simulink model "Batterieersatzschaltbild"  (R2020a)
settings: Solver=VariableStepAuto  StartTime=0.0  StopTime=20  RelTol=1e-3
PreLoadFcn:
  | SubsystemVerbraucherwiderstand = Simulink.Variant('Mode == 1');
  | SubsystemVerbraucherleistung = Simulink.Variant('Mode == 2')
undefined symbols (not defined in the file or in its folder): c_Mo, J_T, L, M_L, Pges, R_A, R_i, Rv, U_b0
settings Model: Creator=ferdi  LastModifiedBy=ferdi

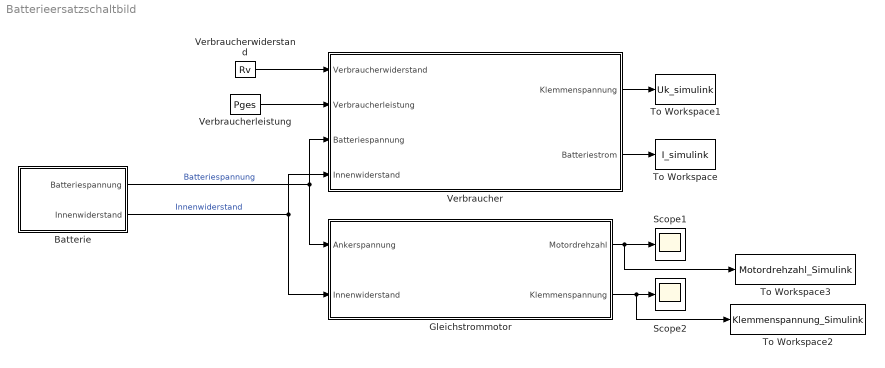
== system Batterieersatzschaltbild ==
  Batterie : Subsystem
      mask Display: image('$imagefile'); % Use "Edit Image" on toolstrip to change.
  Gleichstrommotor : Subsystem
  Scope1 : Scope
  Scope2 : Scope
  To Workspace : ToWorkspace  VariableName=I_simulink  SaveFormat=Timeseries  SampleTime=-1
  To Workspace1 : ToWorkspace  VariableName=Uk_simulink  SaveFormat=Timeseries  SampleTime=-1
  To Workspace2 : ToWorkspace  VariableName=Klemmenspannung_Simulink  SaveFormat=Timeseries  SampleTime=-1
  To Workspace3 : ToWorkspace  VariableName=Motordrehzahl_Simulink  SaveFormat=Timeseries  SampleTime=-1
  Verbraucher : Subsystem  Variant=on
  Verbraucherleistung : Constant  Value=Pges
  Verbraucherwiderstand : Constant  Value=Rv
  wires:
  Gleichstrommotor/1(Motordrehzahl) -> To Workspace3/1, Scope1/1
  Verbraucher/2(Batteriestrom) -> To Workspace/1
  Verbraucher/1(Klemmenspannung) -> To Workspace1/1
  Verbraucherleistung/1 -> Verbraucher/2(Verbraucherleistung)
  Verbraucherwiderstand/1 -> Verbraucher/1(Verbraucherwiderstand)
  Batterie/2(Innenwiderstand) -> Gleichstrommotor/2(Innenwiderstand), Verbraucher/4(Innenwiderstand)  "Innenwiderstand"
  Batterie/1(Batteriespannung) -> Gleichstrommotor/1(Ankerspannung), Verbraucher/3(Batteriespannung)  "Batteriespannung"
  Gleichstrommotor/2(Klemmenspannung) -> To Workspace2/1, Scope2/1

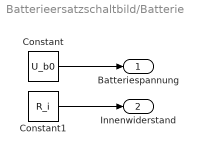
== system Batterieersatzschaltbild/Batterie ==
  Constant : Constant  Value=U_b0
  Constant1 : Constant  Value=R_i
  Batteriespannung : Outport
  Innenwiderstand : Outport  Port=2
  wires:
  Constant/1 -> Batteriespannung/1
  Constant1/1 -> Innenwiderstand/1

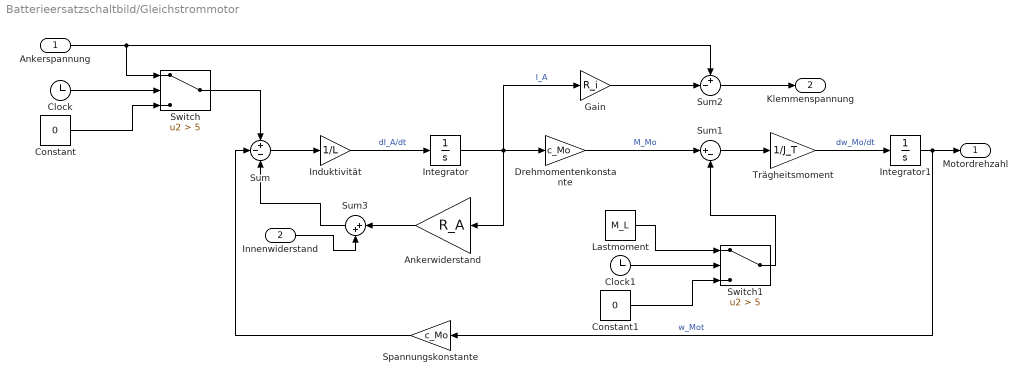
== system Batterieersatzschaltbild/Gleichstrommotor ==
  Ankerspannung : Inport
  Innenwiderstand : Inport  Port=2
  Ankerwiderstand : Gain  Gain=R_A
  Clock : Clock
  Clock1 : Clock
  Constant : Constant  Value=0
  Constant1 : Constant  Value=0
  Drehmomentenkonstante : Gain  Gain=c_Mo
  Gain : Gain  Gain=R_i
  Induktivität : Gain  Gain=1/L
  Integrator : Integrator
  Integrator1 : Integrator
  Lastmoment : Constant  Value=M_L
  Spannungskonstante : Gain  Gain=c_Mo
  Sum : Sum  Inputs=+--
  Sum1 : Sum  Inputs=|+-
  Sum2 : Sum  Inputs=+-|
  Sum3 : Sum  Inputs=|++
  Switch : Switch  Criteria=u2 > Threshold  Threshold=5
  Switch1 : Switch  Criteria=u2 > Threshold  Threshold=5
  Trägheitsmoment : Gain  Gain=1/J_T
  Motordrehzahl : Outport
  Klemmenspannung : Outport  Port=2
  wires:
  Constant/1 -> Switch/3
  Integrator1/1 -> Motordrehzahl/1, Spannungskonstante/1  "w_Mot"
  Drehmomentenkonstante/1 -> Sum1/1  "M_Mo"
  Sum/1 -> Induktivität/1
  Trägheitsmoment/1 -> Integrator1/1  "dw_Mo/dt"
  Switch/1 -> Sum/1
  Ankerspannung/1 -> Switch/1, Sum2/1
  Sum2/1 -> Klemmenspannung/1
  Gain/1 -> Sum2/2
  Clock/1 -> Switch/2
  Lastmoment/1 -> Switch1/1
  Spannungskonstante/1 -> Sum/2
  Induktivität/1 -> Integrator/1  "dI_A/dt"
  Sum1/1 -> Trägheitsmoment/1
  Integrator/1 -> Gain/1, Drehmomentenkonstante/1, Ankerwiderstand/1  "I_A"
  Clock1/1 -> Switch1/2
  Constant1/1 -> Switch1/3
  Switch1/1 -> Sum1/2
  Ankerwiderstand/1 -> Sum3/1
  Sum3/1 -> Sum/3
  Innenwiderstand/1 -> Sum3/2

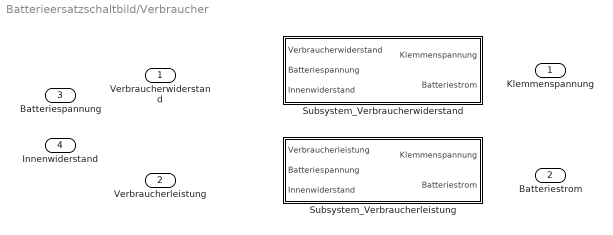
== system Batterieersatzschaltbild/Verbraucher ==
  Verbraucherwiderstand : Inport
  Verbraucherleistung : Inport  Port=2
  Batteriespannung : Inport  Port=3
  Innenwiderstand : Inport  Port=4
  Subsystem_Verbraucherleistung : Subsystem  VariantControl=SubsystemVerbraucherleistung
  Subsystem_Verbraucherwiderstand : Subsystem  VariantControl=SubsystemVerbraucherwiderstand
  Klemmenspannung : Outport
  Batteriestrom : Outport  Port=2

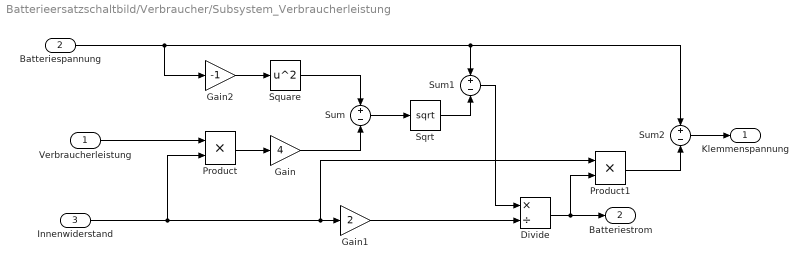
== system Batterieersatzschaltbild/Verbraucher/Subsystem_Verbraucherleistung ==
  Verbraucherleistung : Inport
  Batteriespannung : Inport  Port=2
  Innenwiderstand : Inport  Port=3
  Divide : Product  Inputs=*/
  Gain : Gain  Gain=4
  Gain1 : Gain  Gain=2
  Gain2 : Gain  Gain=-1
  Product : Product
  Product1 : Product
  Sqrt : Sqrt  SaturateOnIntegerOverflow=on
  Square : Math  Operator=square  SaturateOnIntegerOverflow=on
  Sum : Sum  Inputs=+-
  Sum1 : Sum  Inputs=+-
  Sum2 : Sum  Inputs=+-
  Klemmenspannung : Outport
  Batteriestrom : Outport  Port=2
  wires:
  Sum2/1 -> Klemmenspannung/1
  Product1/1 -> Sum2/2
  Sum1/1 -> Divide/1
  Gain1/1 -> Divide/2
  Product/1 -> Gain/1
  Gain/1 -> Sum/2
  Sqrt/1 -> Sum1/2
  Sum/1 -> Sqrt/1
  Square/1 -> Sum/1
  Gain2/1 -> Square/1
  Verbraucherleistung/1 -> Product/1
  Innenwiderstand/1 -> Gain1/1, Product1/1, Product/2
  Batteriespannung/1 -> Sum1/1, Sum2/1, Gain2/1
  Divide/1 -> Batteriestrom/1, Product1/2

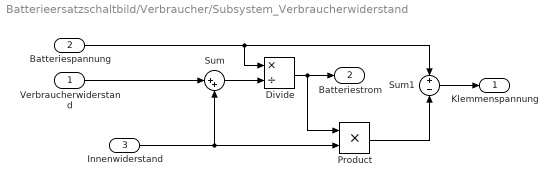
== system Batterieersatzschaltbild/Verbraucher/Subsystem_Verbraucherwiderstand ==
  Verbraucherwiderstand : Inport
  Batteriespannung : Inport  Port=2
  Innenwiderstand : Inport  Port=3
  Divide : Product  Inputs=*/
  Product : Product
  Sum : Sum  Inputs=|++
  Sum1 : Sum  Inputs=+-
  Klemmenspannung : Outport
  Batteriestrom : Outport  Port=2
  wires:
  Innenwiderstand/1 -> Sum/2, Product/2
  Verbraucherwiderstand/1 -> Sum/1
  Divide/1 -> Batteriestrom/1, Product/1
  Sum/1 -> Divide/2
  Sum1/1 -> Klemmenspannung/1
  Product/1 -> Sum1/2
  Batteriespannung/1 -> Divide/1, Sum1/1
